simulink model "ssc_battery_management_R2012b"  (R2014a)
settings: Solver=ode15s  StartTime=0.0  StopTime=2000  FixedStep=0.1  MinStep=1e-10  RelTol=1e-5
PreLoadFcn:
  | ModelPath = fileparts(get_param(bdroot,'FileName'));
  | addpath(ModelPath);
  | 
  | ssc_battery_management_R2012b_ini
values from neighbouring files (symbols this model uses):
  Kt = [0.80,1.10,1.20,1.12;]    [ssc_lead_acid_battery_50Ah_ini.m]    (also in ssc_lead_acid_battery_80Ah_ini.m)
  Kt_Temps = [25 40 60 75]    [ssc_lead_acid_battery_50Ah_ini.m]    (also in ssc_lead_acid_battery_80Ah_ini.m)
  theta_f = -40    [ssc_lead_acid_battery_50Ah_ini.m]    (also in ssc_lead_acid_battery_80Ah_ini.m)
  theta_init = 25    [ssc_lead_acid_battery_50Ah_ini.m]    (also in ssc_lead_acid_battery_80Ah_ini.m)
undefined symbols (not defined in the file or in its folder): AltData100AMaxCurrent, AltData100AVoltage, AltData80AMaxCurrent, AltData80AVoltage, DiscIntNeverNeededParam, sigbuilder_block
undefined symbols (not defined in the file): beta, center, exponent, polyTerms, WendlandNumTerms, width
libraries: fl_lib x146, LeadAcidBattery_lib x36, nesl_utility x28, simulink x1
(part 2 of 4)

== system ssc_battery_management_R2012b/Alternator Variants/Alternator_100A_MBC ==
  Temp : Inport
  RPM : Inport  Port=2
  Alternator : Subsystem
  Controlled Current Source : fl_lib/Electrical/Electrical Sources/Controlled Current Source
  IC : InitialCondition  Value=14.3
  Simulink-PS Converter : nesl_utility/Simulink-PS Converter  PhysicalDomain=network_engine_domain  SubClassName=ps_input  LeftPortType=input  RightPortType=output  PseudoPeriodic=off  Frequencies=[]  NoiseDistribution=none  NoiseParameters=[]  Unit=1  AffineConversion=off  InputFiltering=off  SimscapeFilterOrder=1  InputFilterTimeConstant=.001  UdotUserProvided=0
  Voltage sensor : Subsystem
  + : PMIOPort  Tag=PMCPort  Port=1  Side=Right
  - : PMIOPort  Tag=PMCPort  Port=2  Side=Right
  tag scope: gen_current=global, gen_duty_cycle=global
  wires:
  Temp/1 -> Alternator/1(Temp)  "Temp"
  RPM/1 -> Alternator/2(RPM)  "RPM"
  Alternator/2(Current) -> [gen_current], Simulink-PS Converter/1  "Current"
  Alternator/1(Load Factor) -> [gen_duty_cycle]  "Load Factor"
  [gen_voltage] -> IC/1
  IC/1 -> Alternator/3(Voltage)  "V"
  connections:
  Controlled Current Source/RConn2 -- Voltage sensor/RConn1 -- -/RConn1
  Controlled Current Source/LConn1 -- +/RConn1 -- Voltage sensor/LConn1
  Simulink-PS Converter/RConn1 -- Controlled Current Source/RConn1

== system ssc_battery_management_R2012b/Alternator Variants/Alternator_80A_LUT ==
  Temp : Inport
  RPM : Inport  Port=2
  Alternator : Subsystem
  Controlled Current Source : fl_lib/Electrical/Electrical Sources/Controlled Current Source
  IC : InitialCondition  Value=14.3
  Simulink-PS Converter : nesl_utility/Simulink-PS Converter  PhysicalDomain=network_engine_domain  SubClassName=ps_input  LeftPortType=input  RightPortType=output  PseudoPeriodic=off  Frequencies=[]  NoiseDistribution=none  NoiseParameters=[]  Unit=1  AffineConversion=off  InputFiltering=off  SimscapeFilterOrder=1  InputFilterTimeConstant=.001  UdotUserProvided=0
  Voltage sensor : Subsystem
  + : PMIOPort  Tag=PMCPort  Port=1  Side=Right
  - : PMIOPort  Tag=PMCPort  Port=2  Side=Right
  tag scope: gen_current=global, gen_duty_cycle=global
  wires:
  Temp/1 -> Alternator/1(Temp)  "Temp"
  RPM/1 -> Alternator/2(RPM)  "RPM"
  Alternator/2(Current) -> [gen_current], Simulink-PS Converter/1  "Current"
  Alternator/1(Load Factor) -> [gen_duty_cycle]  "Load Factor"
  [gen_voltage] -> IC/1
  IC/1 -> Alternator/3(Voltage)  "V"
  connections:
  Controlled Current Source/RConn2 -- Voltage sensor/RConn1 -- -/RConn1
  Controlled Current Source/LConn1 -- +/RConn1 -- Voltage sensor/LConn1
  Simulink-PS Converter/RConn1 -- Controlled Current Source/RConn1

== system ssc_battery_management_R2012b/Alternator Variants/Alternator_80A_MBC ==
  Temp : Inport
  RPM : Inport  Port=2
  Alternator : Subsystem
  Controlled Current Source : fl_lib/Electrical/Electrical Sources/Controlled Current Source
  IC : InitialCondition  Value=14.3
  Simulink-PS Converter : nesl_utility/Simulink-PS Converter  PhysicalDomain=network_engine_domain  SubClassName=ps_input  LeftPortType=input  RightPortType=output  PseudoPeriodic=off  Frequencies=[]  NoiseDistribution=none  NoiseParameters=[]  Unit=1  AffineConversion=off  InputFiltering=off  SimscapeFilterOrder=1  InputFilterTimeConstant=.001  UdotUserProvided=0
  Voltage sensor : Subsystem
  + : PMIOPort  Tag=PMCPort  Port=1  Side=Right
  - : PMIOPort  Tag=PMCPort  Port=2  Side=Right
  tag scope: gen_current=global, gen_duty_cycle=global
  wires:
  IC/1 -> Alternator/3(Voltage)  "V"
  [gen_voltage] -> IC/1
  Alternator/1(Load Factor) -> [gen_duty_cycle]  "Load Factor"
  Alternator/2(Current) -> Simulink-PS Converter/1, [gen_current]  "Current"
  RPM/1 -> Alternator/2(RPM)  "RPM"
  Temp/1 -> Alternator/1(Temp)  "Temp"
  connections:
  Simulink-PS Converter/RConn1 -- Controlled Current Source/RConn1
  Voltage sensor/LConn1 -- +/RConn1 -- Controlled Current Source/LConn1
  -/RConn1 -- Voltage sensor/RConn1 -- Controlled Current Source/RConn2

== system ssc_battery_management_R2012b/Lead-Acid Battery/Battery Cell 1 ==
  C1 : LeadAcidBattery_lib/Main Branch Capacitance, C1  Tau1=Tau1 s  Cmin=1e-5 F
  Diode : fl_lib/Electrical/Electrical Elements/Diode  Vf=0.6 V  Ron=0.3 Ohm  Goff=1e-08 1/Ohm  i_specify=off  i_priority=High  i=0 A  v_specify=off  v_priority=High  v=0 V
  Ep : fl_lib/Electrical/Electrical Sources/DC Voltage Source  v0=Ep V
  Main Branch Voltage Source (Em) : LeadAcidBattery_lib/Main Branch Voltage Source, Em  Em0=Emo V  Ke=Ke V/K  Kc=Kc  C0=Costar s*A  Istar=Istar A  delta=delta  Tau1=Tau1 s  Qinit=Qe_init s*A
  R0 : LeadAcidBattery_lib/Terminal Resistance, R0  R00=Roo Ohm  A0=Ao
  R1 : LeadAcidBattery_lib/Main Branch Resistance, R1  R10=R10 Ohm  DOC_min=1e-006
  R2 : LeadAcidBattery_lib/Main Branch Resistance, R2  R20=R20 Ohm  A21=A21  A22=A22  Istar=Istar A
  Rp : LeadAcidBattery_lib/Parasitic Branch Resistance, Rp  Gp0=Gpo 1/Ohm  Vp0=Vpo V  Ap=Ap  Tf=theta_f C
  Thermal Model : Subsystem
  H : PMIOPort  Tag=PMCPort  Port=1  Side=Right
  + : PMIOPort  Tag=PMCPort  Port=2  Side=Left
  - : PMIOPort  Tag=PMCPort  Port=3  Side=Left
  connections:
  Diode/LConn1 -- R0/RConn1 -- R2/LConn2
  R2/RConn2 -- Thermal Model/LConn1
  -/RConn1 -- Ep/RConn1 -- Main Branch Voltage Source (Em)/RConn1
  Thermal Model/RConn1 -- Main Branch Voltage Source (Em)/RConn3
  Diode/RConn1 -- Rp/LConn1
  Ep/LConn1 -- Rp/RConn2
  Thermal Model/LConn2 -- H/RConn1
  R2/LConn1 -- Main Branch Voltage Source (Em)/LConn1 -- R0/LConn1
  R1/LConn2 -- C1/LConn1
  R1/LConn1 -- C1/LConn2 -- R2/RConn1
  Main Branch Voltage Source (Em)/LConn3 -- C1/RConn1 -- R1/RConn2
  Main Branch Voltage Source (Em)/LConn2 -- R1/RConn1
  R0/LConn2 -- +/RConn1
  Thermal Model/RConn2 -- Main Branch Voltage Source (Em)/RConn2 -- Rp/RConn1

== system ssc_battery_management_R2012b/Lead-Acid Battery/Battery Cell 2 ==
  C1 : LeadAcidBattery_lib/Main Branch Capacitance, C1  Tau1=Tau1 s  Cmin=1e-5 F
  Diode : fl_lib/Electrical/Electrical Elements/Diode  Vf=0.6 V  Ron=0.3 Ohm  Goff=1e-08 1/Ohm  i_specify=off  i_priority=High  i=0 A  v_specify=off  v_priority=High  v=0 V
  Ep : fl_lib/Electrical/Electrical Sources/DC Voltage Source  v0=Ep V
  Main Branch Voltage Source (Em) : LeadAcidBattery_lib/Main Branch Voltage Source, Em  Em0=Emo V  Ke=Ke V/K  Kc=Kc  C0=Costar s*A  Istar=Istar A  delta=delta  Tau1=Tau1 s  Qinit=Qe_init s*A
  R0 : LeadAcidBattery_lib/Terminal Resistance, R0  R00=Roo Ohm  A0=Ao
  R1 : LeadAcidBattery_lib/Main Branch Resistance, R1  R10=R10 Ohm  DOC_min=1e-006
  R2 : LeadAcidBattery_lib/Main Branch Resistance, R2  R20=R20 Ohm  A21=A21  A22=A22  Istar=Istar A
  Rp : LeadAcidBattery_lib/Parasitic Branch Resistance, Rp  Gp0=Gpo 1/Ohm  Vp0=Vpo V  Ap=Ap  Tf=theta_f C
  Thermal Model : Subsystem
  H : PMIOPort  Tag=PMCPort  Port=1  Side=Right
  + : PMIOPort  Tag=PMCPort  Port=2  Side=Left
  - : PMIOPort  Tag=PMCPort  Port=3  Side=Left
  connections:
  Rp/RConn1 -- Main Branch Voltage Source (Em)/RConn2 -- Thermal Model/RConn2
  R0/LConn2 -- +/RConn1
  Main Branch Voltage Source (Em)/LConn2 -- R1/RConn1
  R1/RConn2 -- C1/RConn1 -- Main Branch Voltage Source (Em)/LConn3
  R2/RConn1 -- C1/LConn2 -- R1/LConn1
  R1/LConn2 -- C1/LConn1
  R0/LConn1 -- Main Branch Voltage Source (Em)/LConn1 -- R2/LConn1
  Thermal Model/LConn2 -- H/RConn1
  Ep/LConn1 -- Rp/RConn2
  Diode/RConn1 -- Rp/LConn1
  Thermal Model/RConn1 -- Main Branch Voltage Source (Em)/RConn3
  Main Branch Voltage Source (Em)/RConn1 -- Ep/RConn1 -- -/RConn1
  R2/RConn2 -- Thermal Model/LConn1
  R2/LConn2 -- R0/RConn1 -- Diode/LConn1

== system ssc_battery_management_R2012b/Lead-Acid Battery/Battery Cell 3 ==
  C1 : LeadAcidBattery_lib/Main Branch Capacitance, C1  Tau1=Tau1 s  Cmin=1e-5 F
  Diode : fl_lib/Electrical/Electrical Elements/Diode  Vf=0.6 V  Ron=0.3 Ohm  Goff=1e-08 1/Ohm  i_specify=off  i_priority=High  i=0 A  v_specify=off  v_priority=High  v=0 V
  Ep : fl_lib/Electrical/Electrical Sources/DC Voltage Source  v0=Ep V
  Main Branch Voltage Source (Em) : LeadAcidBattery_lib/Main Branch Voltage Source, Em  Em0=Emo V  Ke=Ke V/K  Kc=Kc  C0=Costar s*A  Istar=Istar A  delta=delta  Tau1=Tau1 s  Qinit=Qe_init s*A
  R0 : LeadAcidBattery_lib/Terminal Resistance, R0  R00=Roo Ohm  A0=Ao
  R1 : LeadAcidBattery_lib/Main Branch Resistance, R1  R10=R10 Ohm  DOC_min=1e-006
  R2 : LeadAcidBattery_lib/Main Branch Resistance, R2  R20=R20 Ohm  A21=A21  A22=A22  Istar=Istar A
  Rp : LeadAcidBattery_lib/Parasitic Branch Resistance, Rp  Gp0=Gpo 1/Ohm  Vp0=Vpo V  Ap=Ap  Tf=theta_f C
  Thermal Model : Subsystem
  H : PMIOPort  Tag=PMCPort  Port=1  Side=Right
  + : PMIOPort  Tag=PMCPort  Port=2  Side=Left
  - : PMIOPort  Tag=PMCPort  Port=3  Side=Left
  connections:
  Rp/RConn1 -- Main Branch Voltage Source (Em)/RConn2 -- Thermal Model/RConn2
  R0/LConn2 -- +/RConn1
  Main Branch Voltage Source (Em)/LConn2 -- R1/RConn1
  R1/RConn2 -- C1/RConn1 -- Main Branch Voltage Source (Em)/LConn3
  R2/RConn1 -- C1/LConn2 -- R1/LConn1
  R1/LConn2 -- C1/LConn1
  R0/LConn1 -- Main Branch Voltage Source (Em)/LConn1 -- R2/LConn1
  Thermal Model/LConn2 -- H/RConn1
  Ep/LConn1 -- Rp/RConn2
  Diode/RConn1 -- Rp/LConn1
  Thermal Model/RConn1 -- Main Branch Voltage Source (Em)/RConn3
  Main Branch Voltage Source (Em)/RConn1 -- Ep/RConn1 -- -/RConn1
  R2/RConn2 -- Thermal Model/LConn1
  R2/LConn2 -- R0/RConn1 -- Diode/LConn1

== system ssc_battery_management_R2012b/Lead-Acid Battery/Battery Cell 4 ==
  C1 : LeadAcidBattery_lib/Main Branch Capacitance, C1  Tau1=Tau1 s  Cmin=1e-5 F
  Diode : fl_lib/Electrical/Electrical Elements/Diode  Vf=0.6 V  Ron=0.3 Ohm  Goff=1e-08 1/Ohm  i_specify=off  i_priority=High  i=0 A  v_specify=off  v_priority=High  v=0 V
  Ep : fl_lib/Electrical/Electrical Sources/DC Voltage Source  v0=Ep V
  Main Branch Voltage Source (Em) : LeadAcidBattery_lib/Main Branch Voltage Source, Em  Em0=Emo V  Ke=Ke V/K  Kc=Kc  C0=Costar s*A  Istar=Istar A  delta=delta  Tau1=Tau1 s  Qinit=Qe_init s*A
  R0 : LeadAcidBattery_lib/Terminal Resistance, R0  R00=Roo Ohm  A0=Ao
  R1 : LeadAcidBattery_lib/Main Branch Resistance, R1  R10=R10 Ohm  DOC_min=1e-006
  R2 : LeadAcidBattery_lib/Main Branch Resistance, R2  R20=R20 Ohm  A21=A21  A22=A22  Istar=Istar A
  Rp : LeadAcidBattery_lib/Parasitic Branch Resistance, Rp  Gp0=Gpo 1/Ohm  Vp0=Vpo V  Ap=Ap  Tf=theta_f C
  Thermal Model : Subsystem
  H : PMIOPort  Tag=PMCPort  Port=1  Side=Right
  + : PMIOPort  Tag=PMCPort  Port=2  Side=Left
  - : PMIOPort  Tag=PMCPort  Port=3  Side=Left
  connections:
  Rp/RConn1 -- Main Branch Voltage Source (Em)/RConn2 -- Thermal Model/RConn2
  R0/LConn2 -- +/RConn1
  Main Branch Voltage Source (Em)/LConn2 -- R1/RConn1
  R1/RConn2 -- C1/RConn1 -- Main Branch Voltage Source (Em)/LConn3
  R2/RConn1 -- C1/LConn2 -- R1/LConn1
  R1/LConn2 -- C1/LConn1
  R0/LConn1 -- Main Branch Voltage Source (Em)/LConn1 -- R2/LConn1
  Thermal Model/LConn2 -- H/RConn1
  Ep/LConn1 -- Rp/RConn2
  Diode/RConn1 -- Rp/LConn1
  Thermal Model/RConn1 -- Main Branch Voltage Source (Em)/RConn3
  Main Branch Voltage Source (Em)/RConn1 -- Ep/RConn1 -- -/RConn1
  R2/RConn2 -- Thermal Model/LConn1
  R2/LConn2 -- R0/RConn1 -- Diode/LConn1

== system ssc_battery_management_R2012b/Lead-Acid Battery/Battery Cell 5 ==
  C1 : LeadAcidBattery_lib/Main Branch Capacitance, C1  Tau1=Tau1 s  Cmin=1e-5 F
  Diode : fl_lib/Electrical/Electrical Elements/Diode  Vf=0.6 V  Ron=0.3 Ohm  Goff=1e-08 1/Ohm  i_specify=off  i_priority=High  i=0 A  v_specify=off  v_priority=High  v=0 V
  Ep : fl_lib/Electrical/Electrical Sources/DC Voltage Source  v0=Ep V
  Main Branch Voltage Source (Em) : LeadAcidBattery_lib/Main Branch Voltage Source, Em  Em0=Emo V  Ke=Ke V/K  Kc=Kc  C0=Costar s*A  Istar=Istar A  delta=delta  Tau1=Tau1 s  Qinit=Qe_init s*A
  R0 : LeadAcidBattery_lib/Terminal Resistance, R0  R00=Roo Ohm  A0=Ao
  R1 : LeadAcidBattery_lib/Main Branch Resistance, R1  R10=R10 Ohm  DOC_min=1e-006
  R2 : LeadAcidBattery_lib/Main Branch Resistance, R2  R20=R20 Ohm  A21=A21  A22=A22  Istar=Istar A
  Rp : LeadAcidBattery_lib/Parasitic Branch Resistance, Rp  Gp0=Gpo 1/Ohm  Vp0=Vpo V  Ap=Ap  Tf=theta_f C
  Thermal Model : Subsystem
  H : PMIOPort  Tag=PMCPort  Port=1  Side=Right
  + : PMIOPort  Tag=PMCPort  Port=2  Side=Left
  - : PMIOPort  Tag=PMCPort  Port=3  Side=Left
  connections:
  Rp/RConn1 -- Main Branch Voltage Source (Em)/RConn2 -- Thermal Model/RConn2
  R0/LConn2 -- +/RConn1
  Main Branch Voltage Source (Em)/LConn2 -- R1/RConn1
  R1/RConn2 -- C1/RConn1 -- Main Branch Voltage Source (Em)/LConn3
  R2/RConn1 -- C1/LConn2 -- R1/LConn1
  R1/LConn2 -- C1/LConn1
  R0/LConn1 -- Main Branch Voltage Source (Em)/LConn1 -- R2/LConn1
  Thermal Model/LConn2 -- H/RConn1
  Ep/LConn1 -- Rp/RConn2
  Diode/RConn1 -- Rp/LConn1
  Thermal Model/RConn1 -- Main Branch Voltage Source (Em)/RConn3
  Main Branch Voltage Source (Em)/RConn1 -- Ep/RConn1 -- -/RConn1
  R2/RConn2 -- Thermal Model/LConn1
  R2/LConn2 -- R0/RConn1 -- Diode/LConn1

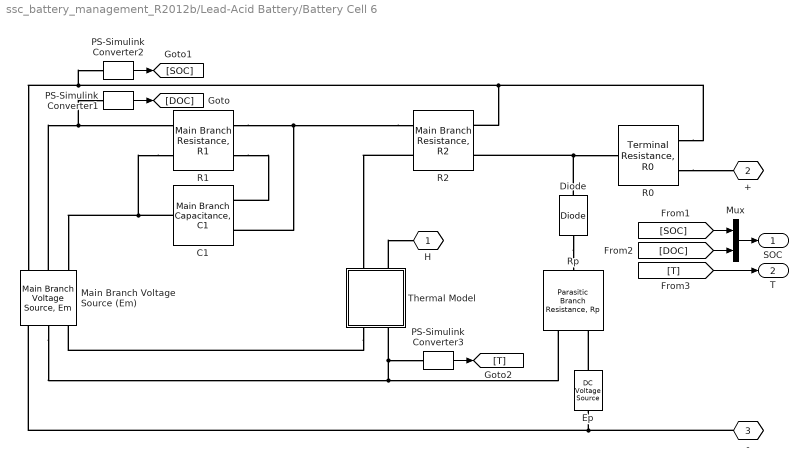
== system ssc_battery_management_R2012b/Lead-Acid Battery/Battery Cell 6 ==
  C1 : LeadAcidBattery_lib/Main Branch Capacitance, C1  Tau1=Tau1 s  Cmin=1e-5 F
  Diode : fl_lib/Electrical/Electrical Elements/Diode  Vf=0.6 V  Ron=0.3 Ohm  Goff=1e-08 1/Ohm  i_specify=off  i_priority=High  i=0 A  v_specify=off  v_priority=High  v=0 V
  Ep : fl_lib/Electrical/Electrical Sources/DC Voltage Source  v0=Ep V
  Main Branch Voltage Source (Em) : LeadAcidBattery_lib/Main Branch Voltage Source, Em  Em0=Emo V  Ke=Ke V/K  Kc=Kc  C0=Costar s*A  Istar=Istar A  delta=delta  Tau1=Tau1 s  Qinit=Qe_init s*A
  Mux : Mux  Inputs=2
  PS-Simulink Converter1 : nesl_utility/PS-Simulink Converter  PhysicalDomain=network_engine_domain  SubClassName=ps_output  LeftPortType=input  RightPortType=output  PseudoPeriodic=off  Frequencies=[]  Unit=1  AffineConversion=off
  PS-Simulink Converter2 : nesl_utility/PS-Simulink Converter  PhysicalDomain=network_engine_domain  SubClassName=ps_output  LeftPortType=input  RightPortType=output  PseudoPeriodic=off  Frequencies=[]  Unit=1  AffineConversion=off
  PS-Simulink Converter3 : nesl_utility/PS-Simulink Converter  PhysicalDomain=network_engine_domain  SubClassName=ps_output  LeftPortType=input  RightPortType=output  PseudoPeriodic=off  Frequencies=[]  Unit=1  AffineConversion=off
  R0 : LeadAcidBattery_lib/Terminal Resistance, R0  R00=Roo Ohm  A0=Ao
  R1 : LeadAcidBattery_lib/Main Branch Resistance, R1  R10=R10 Ohm  DOC_min=1e-006
  R2 : LeadAcidBattery_lib/Main Branch Resistance, R2  R20=R20 Ohm  A21=A21  A22=A22  Istar=Istar A
  Rp : LeadAcidBattery_lib/Parasitic Branch Resistance, Rp  Gp0=Gpo 1/Ohm  Vp0=Vpo V  Ap=Ap  Tf=theta_f C
  Thermal Model : Subsystem
  H : PMIOPort  Tag=PMCPort  Port=1  Side=Right
  + : PMIOPort  Tag=PMCPort  Port=2  Side=Left
  - : PMIOPort  Tag=PMCPort  Port=3  Side=Left
  SOC : Outport
  T : Outport  Port=2
  wires:
  Mux/1 -> SOC/1
  [SOC] -> Mux/1
  [DOC] -> Mux/2
  [T] -> T/1
  PS-Simulink Converter1/1 -> [DOC]
  PS-Simulink Converter2/1 -> [SOC]
  PS-Simulink Converter3/1 -> [T]
  connections:
  Rp/RConn1 -- Main Branch Voltage Source (Em)/RConn2 -- Thermal Model/RConn2 -- PS-Simulink Converter3/LConn1
  R0/LConn2 -- +/RConn1
  Main Branch Voltage Source (Em)/LConn2 -- R1/RConn1 -- PS-Simulink Converter1/LConn1
  R1/RConn2 -- C1/RConn1 -- Main Branch Voltage Source (Em)/LConn3
  R2/RConn1 -- C1/LConn2 -- R1/LConn1
  R1/LConn2 -- C1/LConn1
  R0/LConn1 -- Main Branch Voltage Source (Em)/LConn1 -- PS-Simulink Converter2/LConn1 -- R2/LConn1
  Thermal Model/LConn2 -- H/RConn1
  Ep/LConn1 -- Rp/RConn2
  Diode/RConn1 -- Rp/LConn1
  Thermal Model/RConn1 -- Main Branch Voltage Source (Em)/RConn3
  Main Branch Voltage Source (Em)/RConn1 -- Ep/RConn1 -- -/RConn1
  R2/RConn2 -- Thermal Model/LConn1
  R2/LConn2 -- R0/RConn1 -- Diode/LConn1

== system ssc_battery_management_R2012b/Lead-Acid Battery/Current Sensor ==
  Current Sensor : fl_lib/Electrical/Electrical Sensors/Current Sensor
  PS-Simulink : nesl_utility/PS-Simulink Converter  PhysicalDomain=network_engine_domain  SubClassName=ps_output  LeftPortType=input  RightPortType=output  PseudoPeriodic=off  Frequencies=[]  Unit=A  AffineConversion=off
  + : PMIOPort  Port=1  Side=Left
  - : PMIOPort  Port=2  Side=Right
  tag scope: batt_current=global
  wires:
  PS-Simulink/1 -> [batt_current]
  connections:
  -/RConn1 -- Current Sensor/RConn2
  Current Sensor/LConn1 -- +/RConn1
  Current Sensor/RConn1 -- PS-Simulink/LConn1

== system ssc_battery_management_R2012b/Lead-Acid Battery/Stop if SOC <= 0 ==
  Compare To Zero : simulink/Logic and Bit Operations/Compare To Zero  relop=<=  OutDataTypeStr=boolean  ZeroCross=off
  Stop Simulation : Stop
  wires:
  Compare To Zero/1 -> Stop Simulation/1
  [SOC] -> Compare To Zero/1

== system ssc_battery_management_R2012b/Lead-Acid Battery/Voltage Sensor ==
  PS-Simulink Converter : nesl_utility/PS-Simulink Converter  PhysicalDomain=network_engine_domain  SubClassName=ps_output  LeftPortType=input  RightPortType=output  PseudoPeriodic=off  Frequencies=[]  Unit=V  AffineConversion=off
  Voltage Sensor : fl_lib/Electrical/Electrical Sensors/Voltage Sensor
  + : PMIOPort  Port=1  Side=Left
  - : PMIOPort  Port=2  Side=Right
  tag scope: batt_voltage=global
  wires:
  PS-Simulink Converter/1 -> [batt_voltage]
  connections:
  Voltage Sensor/RConn1 -- PS-Simulink Converter/LConn1
  +/RConn1 -- Voltage Sensor/LConn1
  -/RConn1 -- Voltage Sensor/RConn2

== system ssc_battery_management_R2012b/Alternator Variants/Alternator_100A_LUT/Alternator ==
  Temp : Inport
  RPM : Inport  Port=2
  Voltage : Inport  Port=3
  100A_Max_Current : Lookup_n-D  NumberOfTableDimensions=3  BreakpointsForDimension1=AltData100AMaxCurrent.RPM  BreakpointsForDimension2=AltData100AMaxCurrent.Voltage  BreakpointsForDimension3=AltData100AMaxCurrent.Temp  Table=AltData100AMaxCurrent.Current  InputSameDT=on
  100A_Voltage : Lookup_n-D  NumberOfTableDimensions=3  BreakpointsForDimension1=AltData100AVoltage.RPM  BreakpointsForDimension2=AltData100AVoltage.Current  BreakpointsForDimension3=AltData100AVoltage.Temp  Table=AltData100AVoltage.Voltage  InputSameDT=on
  Product : Product  Inputs=/*  SaturateOnIntegerOverflow=on  OutDataTypeStr=Inherit: Same as first input
  Regulate Voltage : Subsystem
  Saturation1 : Saturate  UpperLimit=inf  LowerLimit=1e-9  ZeroCross=off
  Saturation2 : Saturate  UpperLimit=1  LowerLimit=0  ZeroCross=off
  Saturation3 : Saturate  UpperLimit=15  LowerLimit=13  ZeroCross=off
  Sum : Sum  Inputs=-+|  SaturateOnIntegerOverflow=on
  Load Factor : Outport
  Current : Outport  Port=2
  wires:
  Saturation2/1 -> Load Factor/1
  Saturation1/1 -> Regulate Voltage/1(Max_Current), Product/1  "Max Current"
  Saturation3/1 -> Sum/2  "V_reg"
  Regulate Voltage/1(i) -> Current/1, Product/2, 100A_Voltage/2  "Current"
  Voltage/1 -> Sum/1, 100A_Max_Current/2  "V"
  100A_Max_Current/1 -> Saturation1/1  "Max Current"
  Sum/1 -> Regulate Voltage/2(V error)  "V error"
  100A_Voltage/1 -> Saturation3/1
  RPM/1 -> 100A_Max_Current/1, 100A_Voltage/1  "RPM"
  Temp/1 -> 100A_Max_Current/3, 100A_Voltage/3  "Temp"
  Product/1 -> Saturation2/1

== system ssc_battery_management_R2012b/Alternator Variants/Alternator_100A_LUT/Voltage sensor ==
  PS-Simulink Converter : nesl_utility/PS-Simulink Converter  PhysicalDomain=network_engine_domain  LeftPortType=input  RightPortType=output  SubClassName=ps_output  PseudoPeriodic=off  Frequencies=[]  Unit=V  AffineConversion=off
  Voltage Sensor : fl_lib/Electrical/Electrical Sensors/Voltage Sensor
  + : PMIOPort  Port=1  Side=Left
  - : PMIOPort  Port=2  Side=Right
  tag scope: gen_voltage=global
  wires:
  PS-Simulink Converter/1 -> [gen_voltage]
  connections:
  -/RConn1 -- Voltage Sensor/RConn2
  +/RConn1 -- Voltage Sensor/LConn1
  Voltage Sensor/RConn1 -- PS-Simulink Converter/LConn1

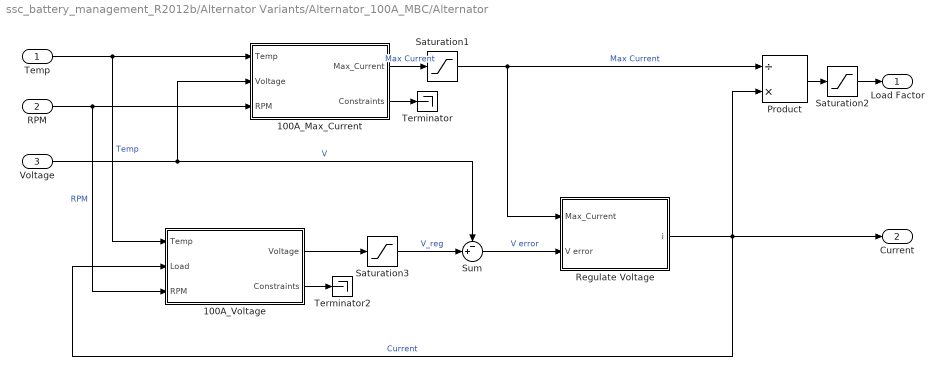
== system ssc_battery_management_R2012b/Alternator Variants/Alternator_100A_MBC/Alternator ==
  Temp : Inport
  RPM : Inport  Port=2
  Voltage : Inport  Port=3
  100A_Max_Current : Subsystem
  100A_Voltage : Subsystem
  Product : Product  Inputs=/*  SaturateOnIntegerOverflow=on  OutDataTypeStr=Inherit: Same as first input
  Regulate Voltage : Subsystem
  Saturation1 : Saturate  UpperLimit=inf  LowerLimit=1e-9  ZeroCross=off
  Saturation2 : Saturate  UpperLimit=1  LowerLimit=0  ZeroCross=off
  Saturation3 : Saturate  UpperLimit=15  LowerLimit=13  ZeroCross=off
  Sum : Sum  Inputs=-+|  SaturateOnIntegerOverflow=on
  Terminator : Terminator
  Terminator2 : Terminator
  Load Factor : Outport
  Current : Outport  Port=2
  wires:
  100A_Max_Current/2(Constraints) -> Terminator/1
  Product/1 -> Saturation2/1
  Temp/1 -> 100A_Voltage/1(Temp), 100A_Max_Current/1(Temp)  "Temp"
  RPM/1 -> 100A_Voltage/3(RPM), 100A_Max_Current/3(RPM)  "RPM"
  100A_Voltage/2(Constraints) -> Terminator2/1
  100A_Voltage/1(Voltage) -> Saturation3/1
  Sum/1 -> Regulate Voltage/2(V error)  "V error"
  100A_Max_Current/1(Max_Current) -> Saturation1/1  "Max Current"
  Voltage/1 -> Sum/1, 100A_Max_Current/2(Voltage)  "V"
  Regulate Voltage/1(i) -> Product/2, Current/1, 100A_Voltage/2(Load)  "Current"
  Saturation3/1 -> Sum/2  "V_reg"
  Saturation1/1 -> Product/1, Regulate Voltage/1(Max_Current)  "Max Current"
  Saturation2/1 -> Load Factor/1

== system ssc_battery_management_R2012b/Alternator Variants/Alternator_100A_MBC/Voltage sensor ==
  PS-Simulink Converter : nesl_utility/PS-Simulink Converter  PhysicalDomain=network_engine_domain  LeftPortType=input  RightPortType=output  SubClassName=ps_output  PseudoPeriodic=off  Frequencies=[]  Unit=V  AffineConversion=off
  Voltage Sensor : fl_lib/Electrical/Electrical Sensors/Voltage Sensor
  + : PMIOPort  Port=1  Side=Left
  - : PMIOPort  Port=2  Side=Right
  tag scope: gen_voltage=global
  wires:
  PS-Simulink Converter/1 -> [gen_voltage]
  connections:
  Voltage Sensor/RConn1 -- PS-Simulink Converter/LConn1
  +/RConn1 -- Voltage Sensor/LConn1
  -/RConn1 -- Voltage Sensor/RConn2

== system ssc_battery_management_R2012b/Alternator Variants/Alternator_80A_LUT/Alternator ==
  Temp : Inport
  RPM : Inport  Port=2
  Voltage : Inport  Port=3
  80A_Max_Current : Lookup_n-D  NumberOfTableDimensions=3  BreakpointsForDimension1=AltData80AMaxCurrent.RPM  BreakpointsForDimension2=AltData80AMaxCurrent.Voltage  BreakpointsForDimension3=AltData80AMaxCurrent.Temp  Table=AltData80AMaxCurrent.Current  InputSameDT=on
  80A_Voltage : Lookup_n-D  NumberOfTableDimensions=3  BreakpointsForDimension1=AltData80AVoltage.RPM  BreakpointsForDimension2=AltData80AVoltage.Current  BreakpointsForDimension3=AltData80AVoltage.Temp  Table=AltData80AVoltage.Voltage  InputSameDT=on
  Product : Product  Inputs=/*  SaturateOnIntegerOverflow=on  OutDataTypeStr=Inherit: Same as first input
  Regulate Voltage : Subsystem
  Saturation1 : Saturate  UpperLimit=inf  LowerLimit=1e-9  ZeroCross=off
  Saturation2 : Saturate  UpperLimit=1  LowerLimit=0  ZeroCross=off
  Saturation3 : Saturate  UpperLimit=15  LowerLimit=13  ZeroCross=off
  Sum : Sum  Inputs=-+|  SaturateOnIntegerOverflow=on
  Load Factor : Outport
  Current : Outport  Port=2
  wires:
  Saturation2/1 -> Load Factor/1
  Product/1 -> Saturation2/1
  Temp/1 -> 80A_Voltage/3, 80A_Max_Current/3  "Temp"
  RPM/1 -> 80A_Voltage/1, 80A_Max_Current/1  "RPM"
  80A_Voltage/1 -> Saturation3/1
  Sum/1 -> Regulate Voltage/2(V error)  "V error"
  80A_Max_Current/1 -> Saturation1/1  "Max Current"
  Voltage/1 -> Sum/1, 80A_Max_Current/2  "V"
  Regulate Voltage/1(i) -> Product/2, Current/1, 80A_Voltage/2  "Current"
  Saturation3/1 -> Sum/2  "V_reg"
  Saturation1/1 -> Product/1, Regulate Voltage/1(Max_Current)  "Max Current"

== system ssc_battery_management_R2012b/Alternator Variants/Alternator_80A_LUT/Voltage sensor ==
  PS-Simulink Converter : nesl_utility/PS-Simulink Converter  PhysicalDomain=network_engine_domain  SubClassName=ps_output  LeftPortType=input  RightPortType=output  PseudoPeriodic=off  Frequencies=[]  Unit=V  AffineConversion=off
  Voltage Sensor : fl_lib/Electrical/Electrical Sensors/Voltage Sensor
  + : PMIOPort  Port=1  Side=Left
  - : PMIOPort  Port=2  Side=Right
  tag scope: gen_voltage=global
  wires:
  PS-Simulink Converter/1 -> [gen_voltage]
  connections:
  Voltage Sensor/RConn1 -- PS-Simulink Converter/LConn1
  +/RConn1 -- Voltage Sensor/LConn1
  -/RConn1 -- Voltage Sensor/RConn2

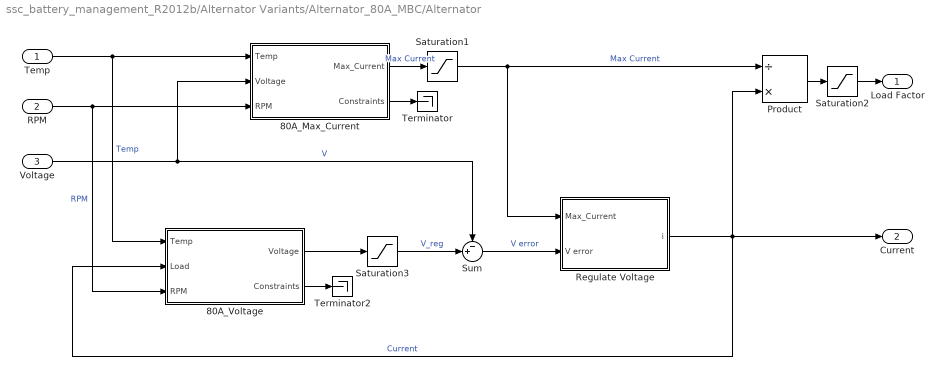
== system ssc_battery_management_R2012b/Alternator Variants/Alternator_80A_MBC/Alternator ==
  Temp : Inport
  RPM : Inport  Port=2
  Voltage : Inport  Port=3
  80A_Max_Current : Subsystem
  80A_Voltage : Subsystem
  Product : Product  Inputs=/*  SaturateOnIntegerOverflow=on  OutDataTypeStr=Inherit: Same as first input
  Regulate Voltage : Subsystem
  Saturation1 : Saturate  UpperLimit=inf  LowerLimit=1e-9  ZeroCross=off
  Saturation2 : Saturate  UpperLimit=1  LowerLimit=0  ZeroCross=off
  Saturation3 : Saturate  UpperLimit=15  LowerLimit=13  ZeroCross=off
  Sum : Sum  Inputs=-+|  SaturateOnIntegerOverflow=on
  Terminator : Terminator
  Terminator2 : Terminator
  Load Factor : Outport
  Current : Outport  Port=2
  wires:
  Saturation1/1 -> Regulate Voltage/1(Max_Current), Product/1  "Max Current"
  Saturation3/1 -> Sum/2  "V_reg"
  Regulate Voltage/1(i) -> Current/1, Product/2, 80A_Voltage/2(Load)  "Current"
  Voltage/1 -> Sum/1, 80A_Max_Current/2(Voltage)  "V"
  80A_Max_Current/1(Max_Current) -> Saturation1/1  "Max Current"
  Sum/1 -> Regulate Voltage/2(V error)  "V error"
  80A_Voltage/1(Voltage) -> Saturation3/1
  80A_Voltage/2(Constraints) -> Terminator2/1
  RPM/1 -> 80A_Max_Current/3(RPM), 80A_Voltage/3(RPM)  "RPM"
  Temp/1 -> 80A_Max_Current/1(Temp), 80A_Voltage/1(Temp)  "Temp"
  Product/1 -> Saturation2/1
  80A_Max_Current/2(Constraints) -> Terminator/1
  Saturation2/1 -> Load Factor/1

== system ssc_battery_management_R2012b/Alternator Variants/Alternator_80A_MBC/Voltage sensor ==
  PS-Simulink Converter : nesl_utility/PS-Simulink Converter  PhysicalDomain=network_engine_domain  LeftPortType=input  RightPortType=output  SubClassName=ps_output  PseudoPeriodic=off  Frequencies=[]  Unit=V  AffineConversion=off
  Voltage Sensor : fl_lib/Electrical/Electrical Sensors/Voltage Sensor
  + : PMIOPort  Port=1  Side=Left
  - : PMIOPort  Port=2  Side=Right
  tag scope: gen_voltage=global
  wires:
  PS-Simulink Converter/1 -> [gen_voltage]
  connections:
  -/RConn1 -- Voltage Sensor/RConn2
  +/RConn1 -- Voltage Sensor/LConn1
  Voltage Sensor/RConn1 -- PS-Simulink Converter/LConn1

== system ssc_battery_management_R2012b/Lead-Acid Battery/Battery Cell 1/Thermal Model ==
  Battery thermal mass : fl_lib/Thermal/Thermal Elements/Thermal Mass  mass=1 kg  sp_heat=Ctheta J/kg/K  Q_specify=off  Q_priority=High  Q=0 J/s  T_specify=on  T_priority=High  T=theta_init+273 K
  Ideal Temperature Sensor : fl_lib/Thermal/Thermal Sensors/Ideal Temperature Sensor
  Ideal Heat Flow Source : fl_lib/Thermal/Thermal Sources/Ideal Heat Flow Source
  Kt as a function of temperature : fl_lib/Physical Signals/Lookup Tables/PS Lookup Table (1D)  x_t=[theta_f, Kt_Temps]+273  y_t=[0 Kt]  interp_method=1  extrap_method=1
  Thermal Reference1 : fl_lib/Thermal/Thermal Elements/Thermal Reference
  Thermal Reference2 : fl_lib/Thermal/Thermal Elements/Thermal Reference
  Ps : PMIOPort  Tag=PMCPort  Port=1  Side=Left
  H : PMIOPort  Tag=PMCPort  Port=2  Side=Left
  Kt : PMIOPort  Tag=PMCPort  Port=3  Side=Right
  T : PMIOPort  Tag=PMCPort  Port=4  Side=Right
  connections:
  Ideal Heat Flow Source/RConn1 -- Ps/RConn1
  Kt/RConn1 -- Kt as a function of temperature/RConn1
  Battery thermal mass/LConn1 -- Ideal Heat Flow Source/LConn1 -- Ideal Temperature Sensor/LConn1 -- H/RConn1
  Thermal Reference1/LConn1 -- Ideal Heat Flow Source/RConn2
  T/RConn1 -- Kt as a function of temperature/LConn1 -- Ideal Temperature Sensor/RConn2
  Ideal Temperature Sensor/RConn1 -- Thermal Reference2/LConn1

== system ssc_battery_management_R2012b/Lead-Acid Battery/Battery Cell 2/Thermal Model ==
  Battery thermal mass : fl_lib/Thermal/Thermal Elements/Thermal Mass  mass=1 kg  sp_heat=Ctheta J/kg/K  Q_specify=off  Q_priority=High  Q=0 J/s  T_specify=on  T_priority=High  T=theta_init+273 K
  Ideal Temperature Sensor : fl_lib/Thermal/Thermal Sensors/Ideal Temperature Sensor
  Ideal Heat Flow Source : fl_lib/Thermal/Thermal Sources/Ideal Heat Flow Source
  Kt as a function of temperature : fl_lib/Physical Signals/Lookup Tables/PS Lookup Table (1D)  x_t=[theta_f, Kt_Temps]+273  y_t=[0 Kt]  interp_method=1  extrap_method=1
  Thermal Reference1 : fl_lib/Thermal/Thermal Elements/Thermal Reference
  Thermal Reference2 : fl_lib/Thermal/Thermal Elements/Thermal Reference
  Ps : PMIOPort  Tag=PMCPort  Port=1  Side=Left
  H : PMIOPort  Tag=PMCPort  Port=2  Side=Left
  Kt : PMIOPort  Tag=PMCPort  Port=3  Side=Right
  T : PMIOPort  Tag=PMCPort  Port=4  Side=Right
  connections:
  Ideal Temperature Sensor/RConn1 -- Thermal Reference2/LConn1
  Ideal Temperature Sensor/RConn2 -- Kt as a function of temperature/LConn1 -- T/RConn1
  Thermal Reference1/LConn1 -- Ideal Heat Flow Source/RConn2
  H/RConn1 -- Ideal Temperature Sensor/LConn1 -- Ideal Heat Flow Source/LConn1 -- Battery thermal mass/LConn1
  Kt/RConn1 -- Kt as a function of temperature/RConn1
  Ideal Heat Flow Source/RConn1 -- Ps/RConn1

== system ssc_battery_management_R2012b/Lead-Acid Battery/Battery Cell 3/Thermal Model ==
  Battery thermal mass : fl_lib/Thermal/Thermal Elements/Thermal Mass  mass=1 kg  sp_heat=Ctheta J/kg/K  Q_specify=off  Q_priority=High  Q=0 J/s  T_specify=on  T_priority=High  T=theta_init+273 K
  Ideal Temperature Sensor : fl_lib/Thermal/Thermal Sensors/Ideal Temperature Sensor
  Ideal Heat Flow Source : fl_lib/Thermal/Thermal Sources/Ideal Heat Flow Source
  Kt as a function of temperature : fl_lib/Physical Signals/Lookup Tables/PS Lookup Table (1D)  x_t=[theta_f, Kt_Temps]+273  y_t=[0 Kt]  interp_method=1  extrap_method=1
  Thermal Reference1 : fl_lib/Thermal/Thermal Elements/Thermal Reference
  Thermal Reference2 : fl_lib/Thermal/Thermal Elements/Thermal Reference
  Ps : PMIOPort  Tag=PMCPort  Port=1  Side=Left
  H : PMIOPort  Tag=PMCPort  Port=2  Side=Left
  Kt : PMIOPort  Tag=PMCPort  Port=3  Side=Right
  T : PMIOPort  Tag=PMCPort  Port=4  Side=Right
  connections:
  Ideal Temperature Sensor/RConn1 -- Thermal Reference2/LConn1
  Ideal Temperature Sensor/RConn2 -- Kt as a function of temperature/LConn1 -- T/RConn1
  Thermal Reference1/LConn1 -- Ideal Heat Flow Source/RConn2
  H/RConn1 -- Ideal Temperature Sensor/LConn1 -- Ideal Heat Flow Source/LConn1 -- Battery thermal mass/LConn1
  Kt/RConn1 -- Kt as a function of temperature/RConn1
  Ideal Heat Flow Source/RConn1 -- Ps/RConn1

== system ssc_battery_management_R2012b/Lead-Acid Battery/Battery Cell 4/Thermal Model ==
  Battery thermal mass : fl_lib/Thermal/Thermal Elements/Thermal Mass  mass=1 kg  sp_heat=Ctheta J/kg/K  Q_specify=off  Q_priority=High  Q=0 J/s  T_specify=on  T_priority=High  T=theta_init+273 K
  Ideal Temperature Sensor : fl_lib/Thermal/Thermal Sensors/Ideal Temperature Sensor
  Ideal Heat Flow Source : fl_lib/Thermal/Thermal Sources/Ideal Heat Flow Source
  Kt as a function of temperature : fl_lib/Physical Signals/Lookup Tables/PS Lookup Table (1D)  x_t=[theta_f, Kt_Temps]+273  y_t=[0 Kt]  interp_method=1  extrap_method=1
  Thermal Reference1 : fl_lib/Thermal/Thermal Elements/Thermal Reference
  Thermal Reference2 : fl_lib/Thermal/Thermal Elements/Thermal Reference
  Ps : PMIOPort  Tag=PMCPort  Port=1  Side=Left
  H : PMIOPort  Tag=PMCPort  Port=2  Side=Left
  Kt : PMIOPort  Tag=PMCPort  Port=3  Side=Right
  T : PMIOPort  Tag=PMCPort  Port=4  Side=Right
  connections:
  Ideal Temperature Sensor/RConn1 -- Thermal Reference2/LConn1
  Ideal Temperature Sensor/RConn2 -- Kt as a function of temperature/LConn1 -- T/RConn1
  Thermal Reference1/LConn1 -- Ideal Heat Flow Source/RConn2
  H/RConn1 -- Ideal Temperature Sensor/LConn1 -- Ideal Heat Flow Source/LConn1 -- Battery thermal mass/LConn1
  Kt/RConn1 -- Kt as a function of temperature/RConn1
  Ideal Heat Flow Source/RConn1 -- Ps/RConn1

== system ssc_battery_management_R2012b/Lead-Acid Battery/Battery Cell 5/Thermal Model ==
  Battery thermal mass : fl_lib/Thermal/Thermal Elements/Thermal Mass  mass=1 kg  sp_heat=Ctheta J/kg/K  Q_specify=off  Q_priority=High  Q=0 J/s  T_specify=on  T_priority=High  T=theta_init+273 K
  Ideal Temperature Sensor : fl_lib/Thermal/Thermal Sensors/Ideal Temperature Sensor
  Ideal Heat Flow Source : fl_lib/Thermal/Thermal Sources/Ideal Heat Flow Source
  Kt as a function of temperature : fl_lib/Physical Signals/Lookup Tables/PS Lookup Table (1D)  x_t=[theta_f, Kt_Temps]+273  y_t=[0 Kt]  interp_method=1  extrap_method=1
  Thermal Reference1 : fl_lib/Thermal/Thermal Elements/Thermal Reference
  Thermal Reference2 : fl_lib/Thermal/Thermal Elements/Thermal Reference
  Ps : PMIOPort  Tag=PMCPort  Port=1  Side=Left
  H : PMIOPort  Tag=PMCPort  Port=2  Side=Left
  Kt : PMIOPort  Tag=PMCPort  Port=3  Side=Right
  T : PMIOPort  Tag=PMCPort  Port=4  Side=Right
  connections:
  Ideal Temperature Sensor/RConn1 -- Thermal Reference2/LConn1
  Ideal Temperature Sensor/RConn2 -- Kt as a function of temperature/LConn1 -- T/RConn1
  Thermal Reference1/LConn1 -- Ideal Heat Flow Source/RConn2
  H/RConn1 -- Ideal Temperature Sensor/LConn1 -- Ideal Heat Flow Source/LConn1 -- Battery thermal mass/LConn1
  Kt/RConn1 -- Kt as a function of temperature/RConn1
  Ideal Heat Flow Source/RConn1 -- Ps/RConn1

== system ssc_battery_management_R2012b/Lead-Acid Battery/Battery Cell 6/Thermal Model ==
  Battery thermal mass : fl_lib/Thermal/Thermal Elements/Thermal Mass  mass=1 kg  sp_heat=Ctheta J/kg/K  Q_specify=off  Q_priority=High  Q=0 J/s  T_specify=on  T_priority=High  T=theta_init+273 K
  Ideal Temperature Sensor : fl_lib/Thermal/Thermal Sensors/Ideal Temperature Sensor
  Ideal Heat Flow Source : fl_lib/Thermal/Thermal Sources/Ideal Heat Flow Source
  Kt as a function of temperature : fl_lib/Physical Signals/Lookup Tables/PS Lookup Table (1D)  x_t=[theta_f, Kt_Temps]+273  y_t=[0 Kt]  interp_method=1  extrap_method=1
  Thermal Reference1 : fl_lib/Thermal/Thermal Elements/Thermal Reference
  Thermal Reference2 : fl_lib/Thermal/Thermal Elements/Thermal Reference
  Ps : PMIOPort  Tag=PMCPort  Port=1  Side=Left
  H : PMIOPort  Tag=PMCPort  Port=2  Side=Left
  Kt : PMIOPort  Tag=PMCPort  Port=3  Side=Right
  T : PMIOPort  Tag=PMCPort  Port=4  Side=Right
  connections:
  Ideal Temperature Sensor/RConn1 -- Thermal Reference2/LConn1
  Ideal Temperature Sensor/RConn2 -- Kt as a function of temperature/LConn1 -- T/RConn1
  Thermal Reference1/LConn1 -- Ideal Heat Flow Source/RConn2
  H/RConn1 -- Ideal Temperature Sensor/LConn1 -- Ideal Heat Flow Source/LConn1 -- Battery thermal mass/LConn1
  Kt/RConn1 -- Kt as a function of temperature/RConn1
  Ideal Heat Flow Source/RConn1 -- Ps/RConn1

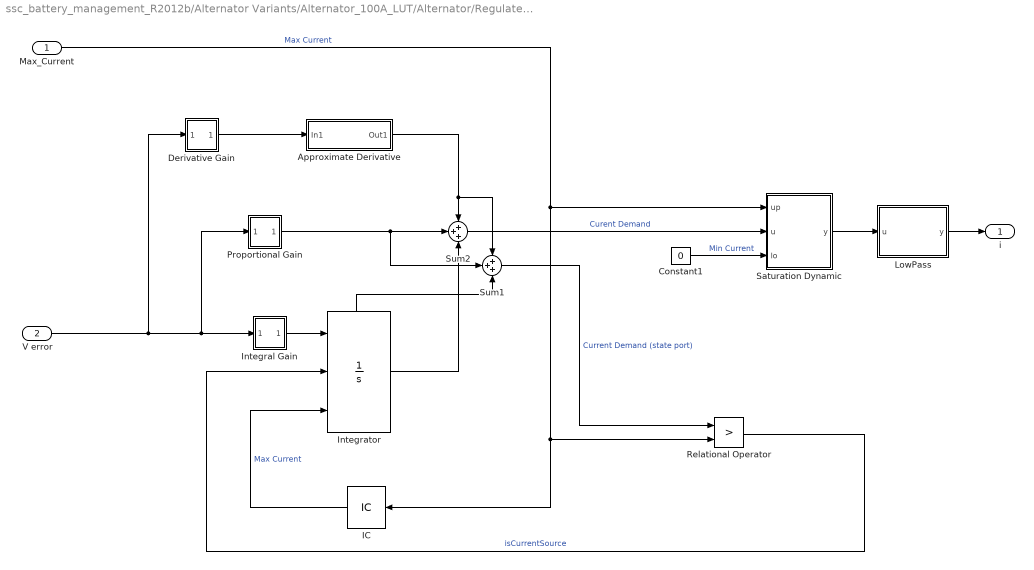
== system ssc_battery_management_R2012b/Alternator Variants/Alternator_100A_LUT/Alternator/Regulate Voltage ==
  Max_Current : Inport
  V error : Inport  Port=2
  Approximate Derivative : Subsystem
  Constant1 : Constant  Value=0  OutDataTypeStr=double
  Derivative Gain : Subsystem  LoadFcn=slideg Load  mask(Slider Gain){low=0, gain=22, high=200}
      settings: CopyFcn=slideg Copy  DeleteFcn=slideg DeleteBlock  NameChangeFcn=slideg NameChange  OpenFcn=slideg Open  CloseFcn=slideg Close  ParentCloseFcn=slideg ParentClose
      mask Display: disp(gain)
  IC : InitialCondition  Value=i_init
  Integral Gain : Subsystem  LoadFcn=slideg Load  mask(Slider Gain){low=0, gain=40, high=200}
      settings: CopyFcn=slideg Copy  DeleteFcn=slideg DeleteBlock  NameChangeFcn=slideg NameChange  OpenFcn=slideg Open  CloseFcn=slideg Close  ParentCloseFcn=slideg ParentClose
      mask Display: disp(gain)
  Integrator : Integrator  ExternalReset=falling  InitialConditionSource=external  LimitOutput=on  UpperSaturationLimit=140  LowerSaturationLimit=0  ShowStatePort=on  IgnoreLimit=on
  LowPass : Subsystem  mask{T=0.3, IC=i_init}
      mask prompts: T "Time Constant"; IC "Initial Condition"
      mask Display:
      | disp(...
      |     strvcat(['1/(' num2str(T) 's+1)'],...
      | ['IC=' num2str(IC)])...
      | )
  Proportional Gain : Subsystem  LoadFcn=slideg Load  mask(Slider Gain){low=0, gain=40, high=200}
      settings: CopyFcn=slideg Copy  DeleteFcn=slideg DeleteBlock  NameChangeFcn=slideg NameChange  OpenFcn=slideg Open  CloseFcn=slideg Close  ParentCloseFcn=slideg ParentClose
      mask Display: disp(gain)
  Relational Operator : RelationalOperator  Operator=>  OutDataTypeStr=boolean
  Saturation Dynamic : Subsystem  mask(Saturation Dynamic){}
      mask help: Bound the range of the second input by using the first input (upper limit) and the third input (lower limit).
      mask Display: plot([0.15 0.85],[.5 .5],[.5 .5],[0.05 0.95],0.15+0.7*[0 .25 .75 1],0.05+0.9*[.25 .25 .75 .75]);
  Sum1 : Sum  Inputs=+++
  Sum2 : Sum  Inputs=+++
  i : Outport
  wires:
  Sum2/1 -> Saturation Dynamic/2(u)  "Curent Demand"
  Proportional Gain/1(Out1) -> Sum2/2, Sum1/2
  Integral Gain/1(Out1) -> Integrator/1
  Integrator/1 -> Sum2/3
  V error/1 -> Integral Gain/1(In1), Proportional Gain/1(In1), Derivative Gain/1(In1)
  Max_Current/1 -> Saturation Dynamic/1(up), Relational Operator/2, IC/1  "Max Current"
  Constant1/1 -> Saturation Dynamic/3(lo)  "Min Current"
  Saturation Dynamic/1(y) -> LowPass/1(u)
  Relational Operator/1 -> Integrator/2  "isCurrentSource"
  IC/1 -> Integrator/3  "Max Current"
  Approximate Derivative/1(Out1) -> Sum2/1, Sum1/1
  Derivative Gain/1(Out1) -> Approximate Derivative/1(In1)
  Integrator/State -> Sum1/3
  Sum1/1 -> Relational Operator/1  "Current Demand (state port)"
  LowPass/1(y) -> i/1

== system ssc_battery_management_R2012b/Alternator Variants/Alternator_100A_MBC/Alternator/100A_Max_Current ==
  Temp : Inport
  Voltage : Inport  Port=2
  RPM : Inport  Port=3
  Constraint Block : Subsystem
  Mx1 : Mux  Inputs=3
  xregrbf : Subsystem
      mask init:
      | xregmaskinitialization;
  Max_Current : Outport
  Constraints : Outport  Port=2
  wires:
  Constraint Block/1(C) -> Constraints/1
  xregrbf/1(Y) -> Max_Current/1
  Mx1/1 -> Constraint Block/1(X), xregrbf/1(X)
  RPM/1 -> Mx1/3
  Voltage/1 -> Mx1/2
  Temp/1 -> Mx1/1

== system ssc_battery_management_R2012b/Alternator Variants/Alternator_100A_MBC/Alternator/100A_Voltage ==
  Temp : Inport
  Load : Inport  Port=2
  RPM : Inport  Port=3
  Constraint Block : Subsystem
  Mx1 : Mux  Inputs=3
  xregrbf : Subsystem
      mask init:
      | xregmaskinitialization;
  Voltage : Outport
  Constraints : Outport  Port=2
  wires:
  Constraint Block/1(C) -> Constraints/1
  xregrbf/1(Y) -> Voltage/1
  Mx1/1 -> Constraint Block/1(X), xregrbf/1(X)
  RPM/1 -> Mx1/3
  Load/1 -> Mx1/2
  Temp/1 -> Mx1/1

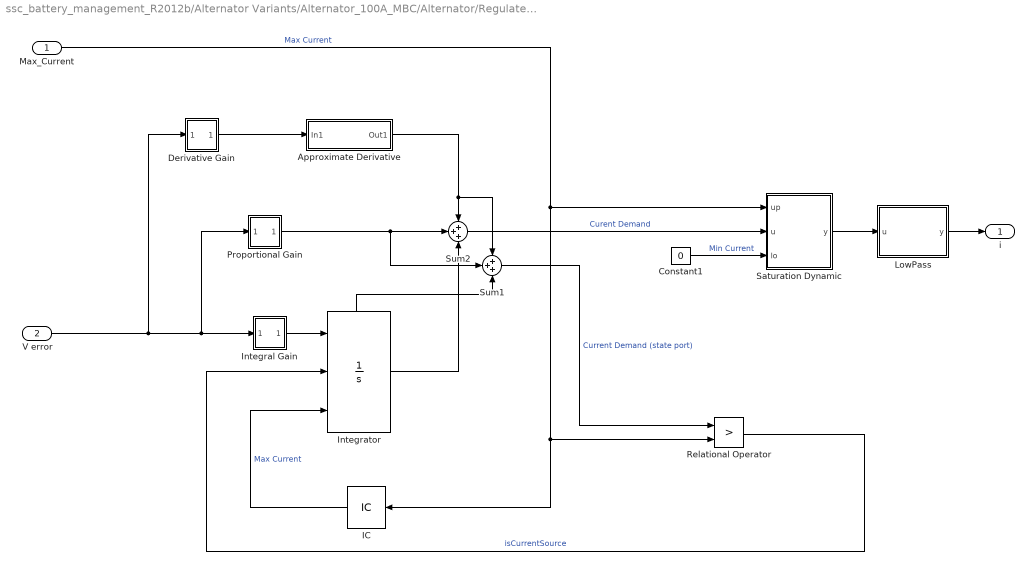
== system ssc_battery_management_R2012b/Alternator Variants/Alternator_100A_MBC/Alternator/Regulate Voltage ==
  Max_Current : Inport
  V error : Inport  Port=2
  Approximate Derivative : Subsystem
  Constant1 : Constant  Value=0  OutDataTypeStr=double
  Derivative Gain : Subsystem  LoadFcn=slideg Load  mask(Slider Gain){low=0, gain=22, high=200}
      settings: CopyFcn=slideg Copy  DeleteFcn=slideg DeleteBlock  NameChangeFcn=slideg NameChange  OpenFcn=slideg Open  CloseFcn=slideg Close  ParentCloseFcn=slideg ParentClose
      mask Display: disp(gain)
  IC : InitialCondition  Value=i_init
  Integral Gain : Subsystem  LoadFcn=slideg Load  mask(Slider Gain){low=0, gain=40, high=200}
      settings: CopyFcn=slideg Copy  DeleteFcn=slideg DeleteBlock  NameChangeFcn=slideg NameChange  OpenFcn=slideg Open  CloseFcn=slideg Close  ParentCloseFcn=slideg ParentClose
      mask Display: disp(gain)
  Integrator : Integrator  ExternalReset=falling  InitialConditionSource=external  LimitOutput=on  UpperSaturationLimit=140  LowerSaturationLimit=0  ShowStatePort=on  IgnoreLimit=on
  LowPass : Subsystem  mask{T=0.3, IC=i_init}
      mask prompts: T "Time Constant"; IC "Initial Condition"
      mask Display:
      | disp(...
      |     strvcat(['1/(' num2str(T) 's+1)'],...
      | ['IC=' num2str(IC)])...
      | )
  Proportional Gain : Subsystem  LoadFcn=slideg Load  mask(Slider Gain){low=0, gain=40, high=200}
      settings: CopyFcn=slideg Copy  DeleteFcn=slideg DeleteBlock  NameChangeFcn=slideg NameChange  OpenFcn=slideg Open  CloseFcn=slideg Close  ParentCloseFcn=slideg ParentClose
      mask Display: disp(gain)
  Relational Operator : RelationalOperator  Operator=>  OutDataTypeStr=boolean
  Saturation Dynamic : Subsystem  mask(Saturation Dynamic){}
      mask help: Bound the range of the second input by using the first input (upper limit) and the third input (lower limit).
      mask Display: plot([0.15 0.85],[.5 .5],[.5 .5],[0.05 0.95],0.15+0.7*[0 .25 .75 1],0.05+0.9*[.25 .25 .75 .75]);
  Sum1 : Sum  Inputs=+++
  Sum2 : Sum  Inputs=+++
  i : Outport
  wires:
  LowPass/1(y) -> i/1
  Sum1/1 -> Relational Operator/1  "Current Demand (state port)"
  Integrator/State -> Sum1/3
  Derivative Gain/1(Out1) -> Approximate Derivative/1(In1)
  Approximate Derivative/1(Out1) -> Sum1/1, Sum2/1
  IC/1 -> Integrator/3  "Max Current"
  Relational Operator/1 -> Integrator/2  "isCurrentSource"
  Saturation Dynamic/1(y) -> LowPass/1(u)
  Constant1/1 -> Saturation Dynamic/3(lo)  "Min Current"
  Max_Current/1 -> IC/1, Relational Operator/2, Saturation Dynamic/1(up)  "Max Current"
  V error/1 -> Derivative Gain/1(In1), Proportional Gain/1(In1), Integral Gain/1(In1)
  Integrator/1 -> Sum2/3
  Integral Gain/1(Out1) -> Integrator/1
  Proportional Gain/1(Out1) -> Sum1/2, Sum2/2
  Sum2/1 -> Saturation Dynamic/2(u)  "Curent Demand"

== system ssc_battery_management_R2012b/Alternator Variants/Alternator_80A_LUT/Alternator/Regulate Voltage ==
  Max_Current : Inport
  V error : Inport  Port=2
  Approximate Derivative : Subsystem
  Constant1 : Constant  Value=0  OutDataTypeStr=double
  Derivative Gain : Subsystem  LoadFcn=slideg Load  mask(Slider Gain){low=0, gain=22, high=200}
      settings: CopyFcn=slideg Copy  DeleteFcn=slideg DeleteBlock  NameChangeFcn=slideg NameChange  OpenFcn=slideg Open  CloseFcn=slideg Close  ParentCloseFcn=slideg ParentClose
      mask Display: disp(gain)
  IC : InitialCondition  Value=i_init
  Integral Gain : Subsystem  LoadFcn=slideg Load  mask(Slider Gain){low=0, gain=40, high=200}
      settings: CopyFcn=slideg Copy  DeleteFcn=slideg DeleteBlock  NameChangeFcn=slideg NameChange  OpenFcn=slideg Open  CloseFcn=slideg Close  ParentCloseFcn=slideg ParentClose
      mask Display: disp(gain)
  Integrator : Integrator  ExternalReset=falling  InitialConditionSource=external  LimitOutput=on  UpperSaturationLimit=140  LowerSaturationLimit=0  ShowStatePort=on  IgnoreLimit=on
  LowPass : Subsystem  mask{T=0.3, IC=i_init}
      mask prompts: T "Time Constant"; IC "Initial Condition"
      mask Display:
      | disp(...
      |     strvcat(['1/(' num2str(T) 's+1)'],...
      | ['IC=' num2str(IC)])...
      | )
  Proportional Gain : Subsystem  LoadFcn=slideg Load  mask(Slider Gain){low=0, gain=40, high=200}
      settings: CopyFcn=slideg Copy  DeleteFcn=slideg DeleteBlock  NameChangeFcn=slideg NameChange  OpenFcn=slideg Open  CloseFcn=slideg Close  ParentCloseFcn=slideg ParentClose
      mask Display: disp(gain)
  Relational Operator : RelationalOperator  Operator=>  OutDataTypeStr=boolean
  Saturation Dynamic : Subsystem  mask(Saturation Dynamic){}
      mask help: Bound the range of the second input by using the first input (upper limit) and the third input (lower limit).
      mask Display: plot([0.15 0.85],[.5 .5],[.5 .5],[0.05 0.95],0.15+0.7*[0 .25 .75 1],0.05+0.9*[.25 .25 .75 .75]);
  Sum1 : Sum  Inputs=+++
  Sum2 : Sum  Inputs=+++
  i : Outport
  wires:
  LowPass/1(y) -> i/1
  Sum1/1 -> Relational Operator/1  "Current Demand (state port)"
  Integrator/State -> Sum1/3
  Derivative Gain/1(Out1) -> Approximate Derivative/1(In1)
  Approximate Derivative/1(Out1) -> Sum1/1, Sum2/1
  IC/1 -> Integrator/3  "Max Current"
  Relational Operator/1 -> Integrator/2  "isCurrentSource"
  Saturation Dynamic/1(y) -> LowPass/1(u)
  Constant1/1 -> Saturation Dynamic/3(lo)  "Min Current"
  Max_Current/1 -> IC/1, Relational Operator/2, Saturation Dynamic/1(up)  "Max Current"
  V error/1 -> Derivative Gain/1(In1), Proportional Gain/1(In1), Integral Gain/1(In1)
  Integrator/1 -> Sum2/3
  Integral Gain/1(Out1) -> Integrator/1
  Proportional Gain/1(Out1) -> Sum1/2, Sum2/2
  Sum2/1 -> Saturation Dynamic/2(u)  "Curent Demand"

== system ssc_battery_management_R2012b/Alternator Variants/Alternator_80A_MBC/Alternator/80A_Max_Current ==
  Temp : Inport
  Voltage : Inport  Port=2
  RPM : Inport  Port=3
  Constraint Block : Subsystem
  Mx1 : Mux  Inputs=3
  xregrbf : Subsystem
      mask init:
      | xregmaskinitialization;
  Max_Current : Outport
  Constraints : Outport  Port=2
  wires:
  Constraint Block/1(C) -> Constraints/1
  xregrbf/1(Y) -> Max_Current/1
  Mx1/1 -> Constraint Block/1(X), xregrbf/1(X)
  RPM/1 -> Mx1/3
  Voltage/1 -> Mx1/2
  Temp/1 -> Mx1/1

== system ssc_battery_management_R2012b/Alternator Variants/Alternator_80A_MBC/Alternator/80A_Voltage ==
  Temp : Inport
  Load : Inport  Port=2
  RPM : Inport  Port=3
  Constraint Block : Subsystem
  Mx1 : Mux  Inputs=3
  xregrbf : Subsystem
      mask init:
      | xregmaskinitialization;
  Voltage : Outport
  Constraints : Outport  Port=2
  wires:
  Constraint Block/1(C) -> Constraints/1
  xregrbf/1(Y) -> Voltage/1
  Mx1/1 -> Constraint Block/1(X), xregrbf/1(X)
  RPM/1 -> Mx1/3
  Load/1 -> Mx1/2
  Temp/1 -> Mx1/1

== system ssc_battery_management_R2012b/Alternator Variants/Alternator_80A_MBC/Alternator/Regulate Voltage ==
  Max_Current : Inport
  V error : Inport  Port=2
  Approximate Derivative : Subsystem
  Constant1 : Constant  Value=0  OutDataTypeStr=double
  Derivative Gain : Subsystem  LoadFcn=slideg Load  mask(Slider Gain){low=0, gain=22, high=200}
      settings: CopyFcn=slideg Copy  DeleteFcn=slideg DeleteBlock  NameChangeFcn=slideg NameChange  OpenFcn=slideg Open  CloseFcn=slideg Close  ParentCloseFcn=slideg ParentClose
      mask Display: disp(gain)
  IC : InitialCondition  Value=i_init
  Integral Gain : Subsystem  LoadFcn=slideg Load  mask(Slider Gain){low=0, gain=40, high=200}
      settings: CopyFcn=slideg Copy  DeleteFcn=slideg DeleteBlock  NameChangeFcn=slideg NameChange  OpenFcn=slideg Open  CloseFcn=slideg Close  ParentCloseFcn=slideg ParentClose
      mask Display: disp(gain)
  Integrator : Integrator  ExternalReset=falling  InitialConditionSource=external  LimitOutput=on  UpperSaturationLimit=140  LowerSaturationLimit=0  ShowStatePort=on  IgnoreLimit=on
  LowPass : Subsystem  mask{T=0.3, IC=i_init}
      mask prompts: T "Time Constant"; IC "Initial Condition"
      mask Display:
      | disp(...
      |     strvcat(['1/(' num2str(T) 's+1)'],...
      | ['IC=' num2str(IC)])...
      | )
  Proportional Gain : Subsystem  LoadFcn=slideg Load  mask(Slider Gain){low=0, gain=40, high=200}
      settings: CopyFcn=slideg Copy  DeleteFcn=slideg DeleteBlock  NameChangeFcn=slideg NameChange  OpenFcn=slideg Open  CloseFcn=slideg Close  ParentCloseFcn=slideg ParentClose
      mask Display: disp(gain)
  Relational Operator : RelationalOperator  Operator=>  OutDataTypeStr=boolean
  Saturation Dynamic : Subsystem  mask(Saturation Dynamic){}
      mask help: Bound the range of the second input by using the first input (upper limit) and the third input (lower limit).
      mask Display: plot([0.15 0.85],[.5 .5],[.5 .5],[0.05 0.95],0.15+0.7*[0 .25 .75 1],0.05+0.9*[.25 .25 .75 .75]);
  Sum1 : Sum  Inputs=+++
  Sum2 : Sum  Inputs=+++
  i : Outport
  wires:
  Sum2/1 -> Saturation Dynamic/2(u)  "Curent Demand"
  Proportional Gain/1(Out1) -> Sum2/2, Sum1/2
  Integral Gain/1(Out1) -> Integrator/1
  Integrator/1 -> Sum2/3
  V error/1 -> Integral Gain/1(In1), Proportional Gain/1(In1), Derivative Gain/1(In1)
  Max_Current/1 -> Saturation Dynamic/1(up), Relational Operator/2, IC/1  "Max Current"
  Constant1/1 -> Saturation Dynamic/3(lo)  "Min Current"
  Saturation Dynamic/1(y) -> LowPass/1(u)
  Relational Operator/1 -> Integrator/2  "isCurrentSource"
  IC/1 -> Integrator/3  "Max Current"
  Approximate Derivative/1(Out1) -> Sum2/1, Sum1/1
  Derivative Gain/1(Out1) -> Approximate Derivative/1(In1)
  Integrator/State -> Sum1/3
  Sum1/1 -> Relational Operator/1  "Current Demand (state port)"
  LowPass/1(y) -> i/1
